simulink model "task1"  (R2024a)
settings: Solver=VariableStepAuto  StartTime=0.0  StopTime=10.0  MaxStep=0.01  RelTol=1e-3
undefined symbols (not defined in the file): A, B, K, x0
settings Model: Creator=sizgr  LastModifiedBy=sizgr

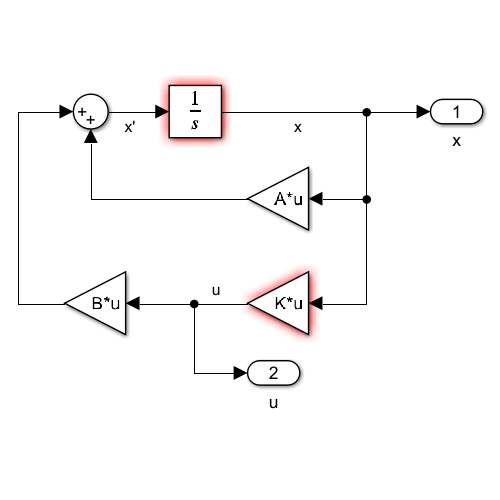
[thumbnail: Simulink's stored preview of the top-level diagram]
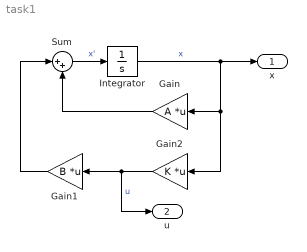
== system task1 ==
  Gain : Gain  Gain=A  Multiplication=Matrix(K*u)
  Gain1 : Gain  Gain=B  Multiplication=Matrix(K*u)
  Gain2 : Gain  Gain=K  Multiplication=Matrix(K*u)
  Integrator : Integrator  InitialCondition=x0
  Sum : Sum  Inputs=|++
  x : Outport
  u : Outport  Port=2
  wires:
  Sum/1 -> Integrator/1  "x'"
  Gain/1 -> Sum/2
  Gain1/1 -> Sum/1
  Gain2/1 -> u/1, Gain1/1  "u"
  Integrator/1 -> x/1, Gain2/1, Gain/1  "x"
